simulink model "MEKF_test_simple"  (R2018b)
settings: Solver=VariableStepAuto  StartTime=0.0  StopTime=50000.0  RelTol=1e-3
libraries: MEKF_SensorCheck_Lib x1
settings Model: Creator=colem  LastModifiedBy=colem

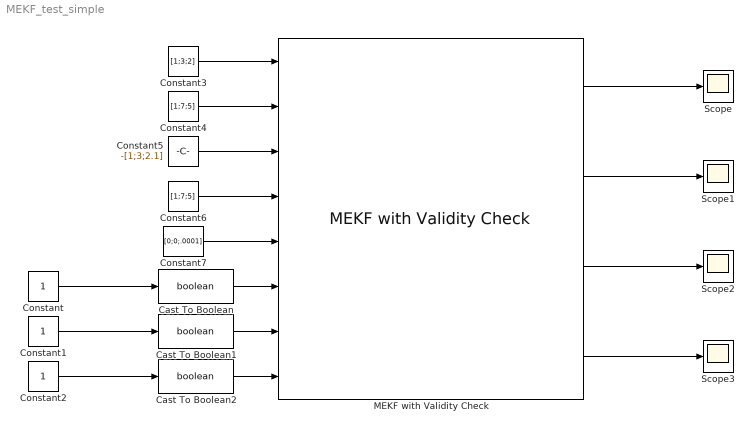
== system MEKF_test_simple ==
  Cast To Boolean : DataTypeConversion  OutDataTypeStr=boolean
  Cast To Boolean1 : DataTypeConversion  OutDataTypeStr=boolean
  Cast To Boolean2 : DataTypeConversion  OutDataTypeStr=boolean
  Constant : Constant
  Constant1 : Constant
  Constant2 : Constant
  Constant3 : Constant  Value=[1;3;2]
  Constant4 : Constant  Value=[1;7;5]
  Constant5 : Constant  Value=-[1;3;2.1]
  Constant6 : Constant  Value=[1;7;5]
  Constant7 : Constant  Value=[0;0;.0001]
  MEKF with Validity Check : MEKF_SensorCheck_Lib/MEKF with Validity Check  SystemSampleTime=-1
      link override "Subsystem Activated if: [All Sensors Valid] or [Gyro Bad and Sun//Mag sensors Valid]/TIME PROPAGATION of Q_EST, COVARIANCE/Constant": Value=fswParams.estimation.dt
      link override "Subsystem Activated if: [Sun//Mag Sensor Invalid and Gyros are Valid] or [Gyro Invalid and Sun//Mag sensors Invalid]/TIME PROPAGATION of Q_EST, COVARIANCE/Constant": Value=fswParams.estimation.dt
  Scope{,1..3} (4 alike) : Scope
  wires:
  Constant/1 -> Cast To Boolean/1
  Constant4/1 -> MEKF with Validity Check/2
  Constant5/1 -> MEKF with Validity Check/3
  Constant6/1 -> MEKF with Validity Check/4
  Constant7/1 -> MEKF with Validity Check/5
  MEKF with Validity Check/1 -> Scope/1
  MEKF with Validity Check/2 -> Scope1/1
  MEKF with Validity Check/3 -> Scope2/1
  MEKF with Validity Check/4 -> Scope3/1
  Constant3/1 -> MEKF with Validity Check/1
  Cast To Boolean/1 -> MEKF with Validity Check/6
  Constant1/1 -> Cast To Boolean1/1
  Cast To Boolean1/1 -> MEKF with Validity Check/7
  Constant2/1 -> Cast To Boolean2/1
  Cast To Boolean2/1 -> MEKF with Validity Check/8
